simulink model "Transmission_Model"  (R2020a)
settings: Solver=VariableStepAuto  StartTime=0.0  StopTime=10.0  RelTol=1e-3
InitFcn:
  | Transmission_Model_init
undefined symbols (not defined in the file): A, B1, B2, C1, D, K, Kr, x0
settings Model: Creator=rizwanahmed  LastModifiedBy=rizwanahmed

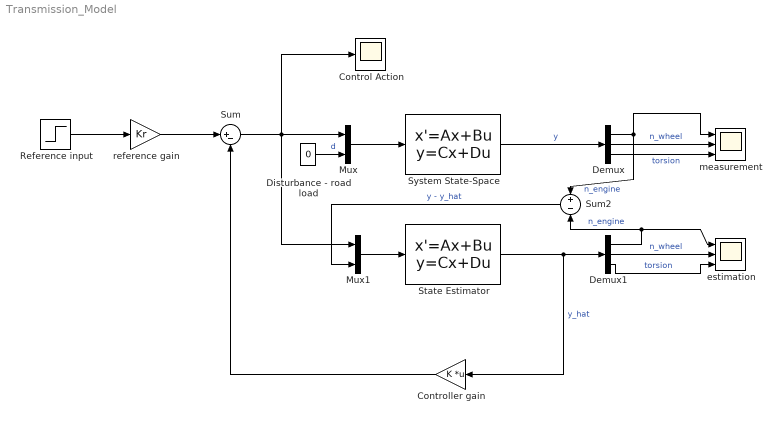
== system Transmission_Model ==
  Control Action : Scope
  Controller gain : Gain  Gain=K  Multiplication=Matrix(K*u)
  Demux : Demux  Outputs=3
  Demux1 : Demux  Outputs=3
  Disturbance - road load : Constant  Value=0
  Mux : Mux  Inputs=2
  Mux1 : Mux  Inputs=2
  Reference input : Step  Time=4  Before=2  After=4  SampleTime=0
  State Estimator : StateSpace  A=A  B=B2  C=C1  D=D  InitialCondition=0
  Sum : Sum  Inputs=|+-
  Sum2 : Sum  Inputs=+-
  System State-Space : StateSpace  A=A  B=B1  C=C1  D=D  InitialCondition=x0
  estimation : Scope  NumInputPorts=3
  measurement : Scope  NumInputPorts=3
  reference gain : Gain  Gain=Kr
  wires:
  State Estimator/1 -> Demux1/1, Controller gain/1  "y_hat"
  Reference input/1 -> reference gain/1
  System State-Space/1 -> Demux/1  "y"
  Demux/1 -> Sum2/1, measurement/1  "n_engine"
  Demux/2 -> measurement/2  "n_wheel"
  Demux/3 -> measurement/3  "torsion"
  Demux1/3 -> estimation/3  "torsion"
  Demux1/2 -> estimation/2  "n_wheel"
  Demux1/1 -> Sum2/2, estimation/1  "n_engine"
  Sum2/1 -> Mux1/2  "y - y_hat"
  Mux/1 -> System State-Space/1
  reference gain/1 -> Sum/1
  Sum/1 -> Control Action/1, Mux1/1, Mux/1
  Controller gain/1 -> Sum/2
  Mux1/1 -> State Estimator/1
  Disturbance - road load/1 -> Mux/2  "d"
